simulink model "velo_id_tc_sl"  (R2019a)
settings: Solver=FixedStepAuto  StartTime=0.0  StopTime=10.0  RelTol=1e-3  EnableMultiTasking=on
values from neighbouring files (symbols this model uses):
  p_const = 0.5    [velo_id_tc.m]    (also in velo_id_verify.m)
  r_const = 1.3    [velo_id_tc.m]    (also in velo_id_verify.m)
  ts = 1/50    (= 0.02)    [sim_init.m]    (also in sim_param.mat; velo_id_tc.m; velo_pi_mdb.m)
  u_ini = 1.5    [velo_id_tc.m]
libraries: arduinolib x2
settings Model: ExtModeTrigDuration=2  Creator=Daichi  LastModifiedBy=Daichi
settings OptimizationCC: EnhancedBackFolding=on  PassReuseOutputArgsAs=Individual arguments  MaxStackSize=64  OptimizeBlockOrder=speed  DifferentSizesBufferReuse=on  OptimizationCustomize=off
settings DebuggingCC: ParameterTunabilityLossMsg=error
settings HardwareCC: ProdBitPerInt=16  ProdBitPerPointer=16  ProdBitPerSizeT=16  ProdBitPerPtrDiffT=16  ProdLargestAtomicFloat=None  ProdWordSize=8  ProdHWDeviceType=Atmel->AVR  UseEmbeddedCoderFeatures=off
settings SFSimCC: MATLABDynamicMemAlloc=off
settings RTWCC: SystemTargetFile=ert.tlc  HardwareBoard=Arduino Mega 2560  TLCOptions=-aInlineSetEventsForThisBaseRateFcn=TLC_FALSE -aSuppressMultiTaskScheduler=TLC_FALSE -aRateBasedStepFcn=1  TemplateMakefile=ert_default_tmf  GenerateReport=on  Toolchain=Arduino AVR  BuildConfiguration=Faster Runs  IncludeHyperlinkInReport=on  LaunchReport=on  GenerateTraceInfo=on  GenerateTraceReport=on  GenerateTraceReportSl=on  GenerateTraceReportSf=on  GenerateTraceReportEml=on
settings CodeAppCC: ForceParamTrailComments=on  IgnoreCustomStorageClasses=off  OperatorAnnotations=on  SimulinkDataObjDesc=on  SFDataObjDesc=on  InsertBlockDesc=on
settings ERTTargetCC: SupportContinuousTime=on  SupportNonInlinedSFcns=on  SupportVariableSizeSignals=on  ExtModeStaticAllocSize=2048

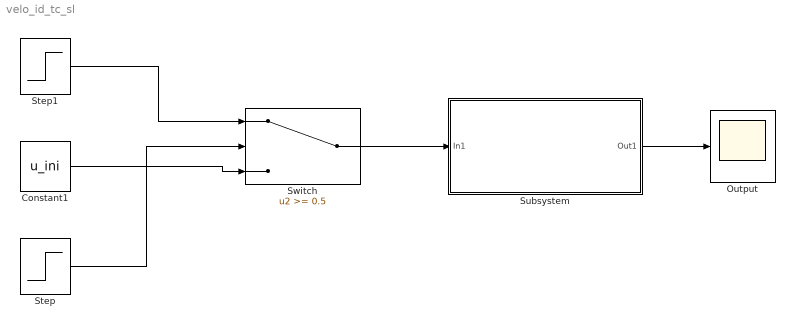
== system velo_id_tc_sl ==
  Constant1 : Constant  Value=u_ini
  Output : Scope
  Step : Step  SampleTime=ts
  Step1 : Step  Before=r_const  After=r_const+p_const  SampleTime=ts
  Subsystem : Subsystem
  Switch : Switch  Threshold=0.5
  wires:
  Step1/1 -> Switch/1
  Constant1/1 -> Switch/3
  Step/1 -> Switch/2
  Switch/1 -> Subsystem/1(In1)
  Subsystem/1(Out1) -> Output/1

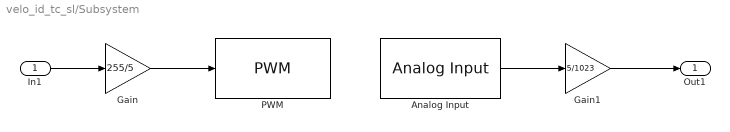
== system velo_id_tc_sl/Subsystem ==
  In1 : Inport
  Analog Input : arduinolib/Analog Input  pinNumber=0  ReadResultsOnly=off  ConversionTriggerSource=Software  ExternalTriggerType=uint32(0)  OutputDataType=uint16  EnableConversionCompleteNotify=off  EnableOuputStatus=off  SampleTime=ts  blockPlatform=arduino
  Gain : Gain  Gain=255/5  OutDataTypeStr=double
  Gain1 : Gain  Gain=5/1023  OutDataTypeStr=double
  PWM : arduinolib/PWM  pinNumber=3  EnableInputFrequency=off  InitialFrequency=2000  InitialDutyCycle=0  NotificationType=None  blockPlatform=arduino
  Out1 : Outport  OutDataTypeStr=double
  wires:
  In1/1 -> Gain/1
  Analog Input/1 -> Gain1/1
  Gain/1 -> PWM/1
  Gain1/1 -> Out1/1
